simulink model "MICRORRED"  (R2018a)
settings: Solver=FixedStepDiscrete  StartTime=0.0  StopTime=0.7  FixedStep=1/(60*32)  RelTol=1e-3  EnableMultiTasking=on
InitFcn:
  | close
  | clear
  | clc
  | Ts=1/(60*32);
  | run script_client_3_inicio_ti.m
  | set_param('MICRORRED/EMISOR-RECEPTOR/TCP_IP_RX3/ESCRITURA', 'Value','0');
  | set_param('MICRORRED/EMISOR-RECEPTOR/TCP_IP_RX3/RETARDO', 'Value','0');
StopFcn:
  | %run script_graficas.m
undefined symbols (not defined in the file or in its folder): DiscIntNeverNeededParam, Int, Ip1, man, Vuc
libraries: powerlib x15, simulink x6, libreria_medidores3 x2, libreria_comunicaciones_red3 x1
(part 2 of 2)

== system MICRORRED/Carga 1 ==
  500 kw3 : powerlib/Elements/Three-Phase Parallel RLC Load  LConnTagsString=A|B|C  Configuration=Y (grounded)  NominalVoltage=13200  Vabc=[1e3 1e3 1e3]  Vabcp=[1e3 1e3 1e3]  NominalFrequency=60  UnbalancedPower=off  ActivePower=500e3  InductivePower=100e3  CapacitivePower=0  Pabc=[10e3 9e3 11e3]  QLabc=[100 90 110]  QCabc=[100 90 110]  Pabcp=[10e3 9e3 11e3]  QLabcp=[100 90 110]  QCabcp=[100 90 110]  Measurements=None  LoadType=constant Z
  a : PMIOPort  Side=Left
  b : PMIOPort  Port=2  Side=Left
  c : PMIOPort  Port=3  Side=Left
  connections:
  500 kw3/LConn1 -- a/RConn1
  500 kw3/LConn3 -- c/RConn1
  500 kw3/LConn2 -- b/RConn1

== system MICRORRED/Carga 2 ==
  500 kw3 : powerlib/Elements/Three-Phase Parallel RLC Load  LConnTagsString=A|B|C  Configuration=Y (grounded)  NominalVoltage=13200  Vabc=[1e3 1e3 1e3]  Vabcp=[1e3 1e3 1e3]  NominalFrequency=60  UnbalancedPower=off  ActivePower=500e3  InductivePower=100e3  CapacitivePower=0  Pabc=[10e3 9e3 11e3]  QLabc=[100 90 110]  QCabc=[100 90 110]  Pabcp=[10e3 9e3 11e3]  QLabcp=[100 90 110]  QCabcp=[100 90 110]  Measurements=None  LoadType=constant Z
  a : PMIOPort  Side=Left
  b : PMIOPort  Port=2  Side=Left
  c : PMIOPort  Port=3  Side=Left
  connections:
  500 kw3/LConn3 -- c/RConn1
  500 kw3/LConn2 -- b/RConn1
  a/RConn1 -- 500 kw3/LConn1

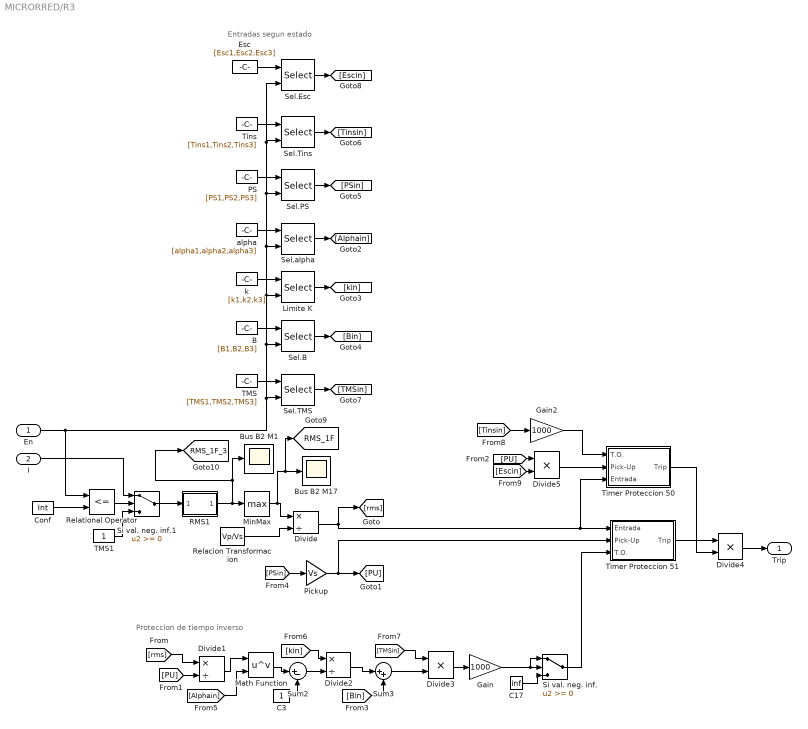
== system MICRORRED/R3 ==
  note: Proteccion de tiempo inverso
  note: Entradas segun estado
  En : Inport
  I : Inport  Port=2
  B : Constant  Value=[B1,B2,B3]
  Bus B2 M1 : Scope
  Bus B2 M17 : Scope
  C17 : Constant  Value=inf
  C3 : Constant
  Conf : Constant  Value=Int
  Divide : Product  Inputs=*/
  Divide1 : Product  Inputs=*/
  Divide2 : Product  Inputs=*/
  Divide3 : Product  Inputs=**
  Divide4 : Product  Inputs=**
  Divide5 : Product  Inputs=**
  Esc : Constant  Value=[Esc1,Esc2,Esc3]
  Gain : Gain  Gain=1000
  Gain2 : Gain  Gain=1000
  Limite K : Selector  InputPortWidth=3  IndexOptions=Index vector (port)  Indices=[1 2 3]  OutputSizes=1
  Math Function : Math  Operator=pow  SaturateOnIntegerOverflow=on
  MinMax : MinMax  Function=max
  PS : Constant  Value=[PS1,PS2,PS3]
  Pickup : Gain  Gain=Vs
  RMS1 : Subsystem
  Relacion Transformacion : Constant  Value=Vp/Vs
  Relational Operator : RelationalOperator  Operator=<=  OutDataTypeStr=boolean  RndMeth=Simplest
  Sel.B : Selector  InputPortWidth=3  IndexOptions=Index vector (port)  Indices=[1 2 3]  OutputSizes=1
  Sel.Esc : Selector  InputPortWidth=3  IndexOptions=Index vector (port)  Indices=[1 2 3]  OutputSizes=1
  Sel.PS : Selector  InputPortWidth=3  IndexOptions=Index vector (port)  Indices=[1 2 3]  OutputSizes=1
  Sel.TMS : Selector  InputPortWidth=3  IndexOptions=Index vector (port)  Indices=[1 2 3]  OutputSizes=1
  Sel.Tins : Selector  InputPortWidth=3  IndexOptions=Index vector (port)  Indices=[1 2 3]  OutputSizes=1
  Sel.alpha : Selector  InputPortWidth=3  IndexOptions=Index vector (port)  Indices=[1 2 3]  OutputSizes=1
  Si val. neg. inf. : Switch
  Si val. neg. inf.1 : Switch
  Sum2 : Sum  Inputs=|+-
  Sum3 : Sum  Inputs=|++
  TMS : Constant  Value=[TMS1,TMS2,TMS3]
  TMS1 : Constant
  Timer Proteccion 50 : Subsystem
  Timer Proteccion 51 : Subsystem
  Tins : Constant  Value=[Tins1,Tins2,Tins3]
  alpha : Constant  Value=[alpha1,alpha2,alpha3]
  k : Constant  Value=[k1,k2,k3]
  Trip : Outport
  tag scope: RMS_1F=global, RMS_1F_3=global
  wires:
  En/1 -> Relational Operator/1, Sel.TMS/2, Sel.B/2, Limite K/2, Sel.alpha/2, Sel.PS/2, Sel.Tins/2, Sel.Esc/2
  Divide4/1 -> Trip/1
  Tins/1 -> Sel.Tins/1
  [Escin] -> Divide5/2
  Sel.Esc/1 -> [Escin]
  C17/1 -> Si val. neg. inf./3
  Esc/1 -> Sel.Esc/1
  Math Function/1 -> Sum2/1
  [kin] -> Divide2/1
  Timer Proteccion 50/1(Trip) -> Divide4/2
  [PSin] -> Pickup/1
  Si val. neg. inf./1 -> Timer Proteccion 51/3(T.O.)
  Sel.TMS/1 -> [TMSin]
  PS/1 -> Sel.PS/1
  [Tinsin] -> Gain2/1
  Timer Proteccion 51/1(Trip) -> Divide4/1
  [Alphain] -> Math Function/2
  Divide3/1 -> Gain/1
  [PU] -> Divide1/2
  [PU] -> Divide5/1
  B/1 -> Sel.B/1
  Divide5/1 -> Timer Proteccion 50/2(Pick-Up)
  Divide2/1 -> Sum3/1
  Gain2/1 -> Timer Proteccion 50/1(T.O.)
  Gain/1 -> Si val. neg. inf./1, Si val. neg. inf./2
  Sum3/1 -> Divide3/2
  Sel.alpha/1 -> [Alphain]
  [Bin] -> Sum3/2
  Relacion Transformacion/1 -> Divide/2
  Divide/1 -> Timer Proteccion 51/1(Entrada), Timer Proteccion 50/3(Entrada), [rms]
  Sum2/1 -> Divide2/2
  Divide1/1 -> Math Function/1
  Limite K/1 -> [kin]
  [rms] -> Divide1/1
  Pickup/1 -> Timer Proteccion 51/2(Pick-Up), [PU]
  Sel.B/1 -> [Bin]
  Sel.PS/1 -> [PSin]
  MinMax/1 -> [RMS_1F], Bus B2 M17/1, Divide/1
  RMS1/1(Out1) -> [RMS_1F_3], Bus B2 M1/1, MinMax/1
  [TMSin] -> Divide3/1
  TMS/1 -> Sel.TMS/1
  C3/1 -> Sum2/2
  k/1 -> Limite K/1
  alpha/1 -> Sel.alpha/1
  Sel.Tins/1 -> [Tinsin]
  I/1 -> Si val. neg. inf.1/1
  Relational Operator/1 -> Si val. neg. inf.1/2
  Si val. neg. inf.1/1 -> RMS1/1(In1)
  Conf/1 -> Relational Operator/2
  TMS1/1 -> Si val. neg. inf.1/3

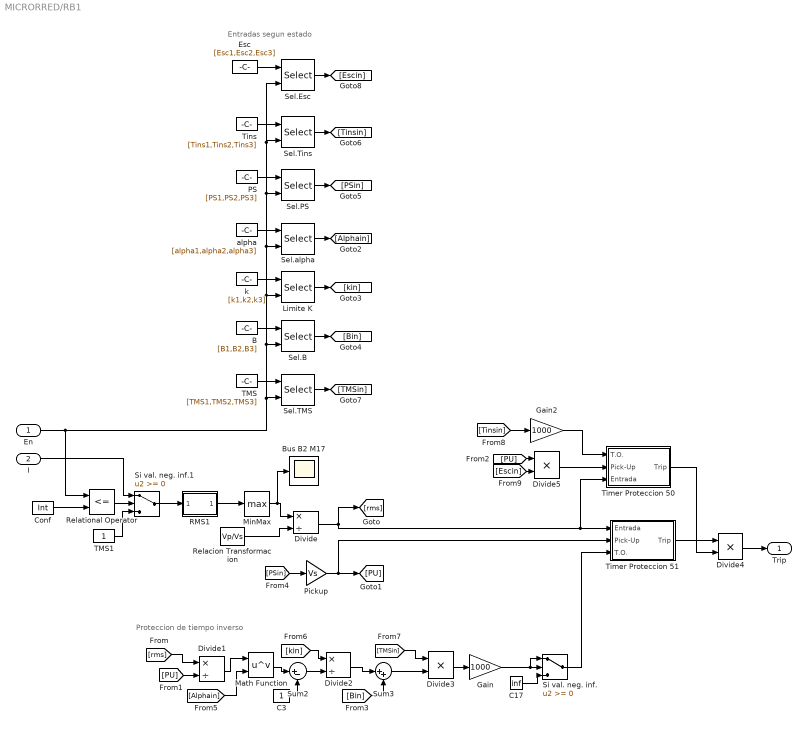
== system MICRORRED/RB1 ==
  note: Entradas segun estado
  note: Proteccion de tiempo inverso
  En : Inport
  I : Inport  Port=2
  B : Constant  Value=[B1,B2,B3]
  Bus B2 M17 : Scope
  C17 : Constant  Value=inf
  C3 : Constant
  Conf : Constant  Value=Int
  Divide : Product  Inputs=*/
  Divide1 : Product  Inputs=*/
  Divide2 : Product  Inputs=*/
  Divide3 : Product  Inputs=**
  Divide4 : Product  Inputs=**
  Divide5 : Product  Inputs=**
  Esc : Constant  Value=[Esc1,Esc2,Esc3]
  Gain : Gain  Gain=1000
  Gain2 : Gain  Gain=1000
  Limite K : Selector  InputPortWidth=3  IndexOptions=Index vector (port)  Indices=[1 2 3]  OutputSizes=1
  Math Function : Math  Operator=pow  SaturateOnIntegerOverflow=on
  MinMax : MinMax  Function=max
  PS : Constant  Value=[PS1,PS2,PS3]
  Pickup : Gain  Gain=Vs
  RMS1 : Subsystem
  Relacion Transformacion : Constant  Value=Vp/Vs
  Relational Operator : RelationalOperator  Operator=<=  OutDataTypeStr=boolean  RndMeth=Simplest
  Sel.B : Selector  InputPortWidth=3  IndexOptions=Index vector (port)  Indices=[1 2 3]  OutputSizes=1
  Sel.Esc : Selector  InputPortWidth=3  IndexOptions=Index vector (port)  Indices=[1 2 3]  OutputSizes=1
  Sel.PS : Selector  InputPortWidth=3  IndexOptions=Index vector (port)  Indices=[1 2 3]  OutputSizes=1
  Sel.TMS : Selector  InputPortWidth=3  IndexOptions=Index vector (port)  Indices=[1 2 3]  OutputSizes=1
  Sel.Tins : Selector  InputPortWidth=3  IndexOptions=Index vector (port)  Indices=[1 2 3]  OutputSizes=1
  Sel.alpha : Selector  InputPortWidth=3  IndexOptions=Index vector (port)  Indices=[1 2 3]  OutputSizes=1
  Si val. neg. inf. : Switch
  Si val. neg. inf.1 : Switch
  Sum2 : Sum  Inputs=|+-
  Sum3 : Sum  Inputs=|++
  TMS : Constant  Value=[TMS1,TMS2,TMS3]
  TMS1 : Constant
  Timer Proteccion 50 : Subsystem
  Timer Proteccion 51 : Subsystem
  Tins : Constant  Value=[Tins1,Tins2,Tins3]
  alpha : Constant  Value=[alpha1,alpha2,alpha3]
  k : Constant  Value=[k1,k2,k3]
  Trip : Outport
  wires:
  TMS1/1 -> Si val. neg. inf.1/3
  Conf/1 -> Relational Operator/2
  Si val. neg. inf.1/1 -> RMS1/1(In1)
  Relational Operator/1 -> Si val. neg. inf.1/2
  I/1 -> Si val. neg. inf.1/1
  Sel.Tins/1 -> [Tinsin]
  alpha/1 -> Sel.alpha/1
  k/1 -> Limite K/1
  C3/1 -> Sum2/2
  TMS/1 -> Sel.TMS/1
  [TMSin] -> Divide3/1
  RMS1/1(Out1) -> MinMax/1
  MinMax/1 -> Divide/1, Bus B2 M17/1
  Sel.PS/1 -> [PSin]
  Sel.B/1 -> [Bin]
  Pickup/1 -> [PU], Timer Proteccion 51/2(Pick-Up)
  [rms] -> Divide1/1
  Limite K/1 -> [kin]
  Divide1/1 -> Math Function/1
  Sum2/1 -> Divide2/2
  Divide/1 -> [rms], Timer Proteccion 50/3(Entrada), Timer Proteccion 51/1(Entrada)
  Relacion Transformacion/1 -> Divide/2
  [Bin] -> Sum3/2
  Sel.alpha/1 -> [Alphain]
  Sum3/1 -> Divide3/2
  Gain/1 -> Si val. neg. inf./2, Si val. neg. inf./1
  Gain2/1 -> Timer Proteccion 50/1(T.O.)
  Divide2/1 -> Sum3/1
  Divide5/1 -> Timer Proteccion 50/2(Pick-Up)
  B/1 -> Sel.B/1
  [PU] -> Divide5/1
  [PU] -> Divide1/2
  Divide3/1 -> Gain/1
  [Alphain] -> Math Function/2
  Timer Proteccion 51/1(Trip) -> Divide4/1
  [Tinsin] -> Gain2/1
  PS/1 -> Sel.PS/1
  Sel.TMS/1 -> [TMSin]
  Si val. neg. inf./1 -> Timer Proteccion 51/3(T.O.)
  [PSin] -> Pickup/1
  Timer Proteccion 50/1(Trip) -> Divide4/2
  [kin] -> Divide2/1
  Math Function/1 -> Sum2/1
  Esc/1 -> Sel.Esc/1
  C17/1 -> Si val. neg. inf./3
  Sel.Esc/1 -> [Escin]
  [Escin] -> Divide5/2
  Tins/1 -> Sel.Tins/1
  Divide4/1 -> Trip/1
  En/1 -> Sel.Esc/2, Sel.Tins/2, Sel.PS/2, Sel.alpha/2, Limite K/2, Sel.B/2, Sel.TMS/2, Relational Operator/1

== system MICRORRED/Subsystem ==
  Trigger : TriggerPort  VariantControl=Variant  ShowOutputPort=on  OutputDataType=double  InitialTriggerSignalState=positive  PortDimensions=1
  Display : Display
  Out1 : Outport
  wires:
  Trigger/1 -> Display/1, Out1/1

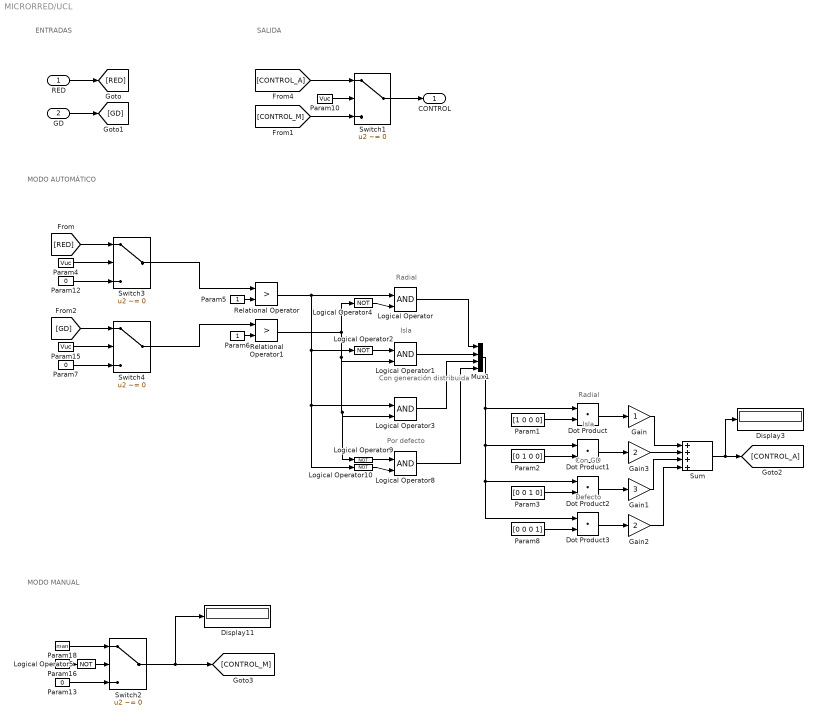
== system MICRORRED/UCL ==
  note: ENTRADAS
  note: Con generación
      | distribuida
  note: Isla
  note: Radial
  note: SALIDA
  note: MODO AUTOMÁTICO
  note: MODO MANUAL
  note: Radial
  note: Isla
  note: Con GD
  note: Por defecto
  note: Defecto
  RED : Inport
  GD : Inport  Port=2
  Display11 : Display
  Display3 : Display
  Dot Product{,1..3} (4 alike) : DotProduct  InputSameDT=on  OutDataTypeStr=Inherit: Inherit via internal rule
  Gain : Gain
  Gain1 : Gain  Gain=3
  Gain2 : Gain  Gain=2
  Gain3 : Gain  Gain=2
  Logical Operator{,1,3,8} (4 alike) : Logic  IconShape=distinctive  AllPortsSameDT=off  OutDataTypeStr=boolean
  Logical Operator{2,4..5,9..10} (5 alike) : Logic  Operator=NOT  AllPortsSameDT=off  OutDataTypeStr=boolean
  Mux1 : Mux
  Param1 : Constant  Value=[1 0 0 0]  OutDataTypeStr=boolean
  Param{4,10,15..16} (4 alike) : Constant  Value=Vuc
  Param12 : Constant  Value=0
  Param13 : Constant  Value=0
  Param18 : Constant  Value=man
  Param2 : Constant  Value=[0 1 0 0]  OutDataTypeStr=boolean
  Param3 : Constant  Value=[0 0 1 0]  OutDataTypeStr=boolean
  Param5 : Constant
  Param6 : Constant
  Param7 : Constant  Value=0
  Param8 : Constant  Value=[0 0 0 1]  OutDataTypeStr=boolean
  Relational Operator : RelationalOperator  Operator=>  OutDataTypeStr=boolean  RndMeth=Nearest
  Relational Operator1 : RelationalOperator  Operator=>  OutDataTypeStr=boolean  RndMeth=Nearest
  Sum : Sum  Inputs=+|+|+|+
  Switch{1..4} (4 alike) : Switch  Criteria=u2 ~= 0
  CONTROL : Outport
  wires:
  Relational Operator/1 -> Logical Operator10/1, Logical Operator3/1, Logical Operator2/1, Logical Operator/1
  Param6/1 -> Relational Operator1/2
  Param5/1 -> Relational Operator/2
  Logical Operator2/1 -> Logical Operator1/1
  Logical Operator4/1 -> Logical Operator/2
  Logical Operator/1 -> Mux1/1
  Logical Operator1/1 -> Mux1/2
  Logical Operator3/1 -> Mux1/3
  Param1/1 -> Dot Product/2
  Dot Product/1 -> Gain/1
  Param2/1 -> Dot Product1/2
  Param3/1 -> Dot Product2/2
  Dot Product1/1 -> Gain3/1
  Dot Product2/1 -> Gain1/1
  Gain/1 -> Sum/1
  Logical Operator5/1 -> Switch2/2
  RED/1 -> [RED]
  Param18/1 -> Switch2/1
  GD/1 -> [GD]
  [RED] -> Switch3/1
  Param12/1 -> Switch3/3
  [GD] -> Switch4/1
  Param7/1 -> Switch4/3
  Param13/1 -> Switch2/3
  Param4/1 -> Switch3/2
  Param15/1 -> Switch4/2
  Param16/1 -> Logical Operator5/1
  Switch2/1 -> [CONTROL_M], Display11/1
  Gain3/1 -> Sum/2
  Gain1/1 -> Sum/3
  Sum/1 -> [CONTROL_A], Display3/1
  Switch3/1 -> Relational Operator/1
  Switch4/1 -> Relational Operator1/1
  Logical Operator9/1 -> Logical Operator8/1
  Logical Operator10/1 -> Logical Operator8/2
  Relational Operator1/1 -> Logical Operator4/1, Logical Operator9/1, Logical Operator3/2, Logical Operator1/2
  Logical Operator8/1 -> Mux1/4
  Param8/1 -> Dot Product3/2
  Mux1/1 -> Dot Product3/1, Dot Product2/1, Dot Product1/1, Dot Product/1
  Dot Product3/1 -> Gain2/1
  Gain2/1 -> Sum/4
  [CONTROL_A] -> Switch1/1
  [CONTROL_M] -> Switch1/3
  Param10/1 -> Switch1/2
  Switch1/1 -> CONTROL/1

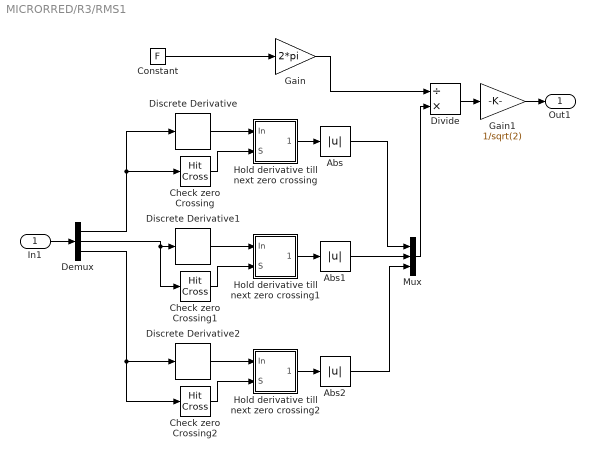
== system MICRORRED/R3/RMS1 ==
  In1 : Inport
  Abs : Abs
  Abs1 : Abs
  Abs2 : Abs
  Check zero Crossing : HitCross
  Check zero Crossing1 : HitCross
  Check zero Crossing2 : HitCross
  Constant : Constant  Value=F
  Demux : Demux  Outputs=3
  Discrete Derivative : simulink/Discrete/Discrete Derivative  gainval=1.0  ICPrevScaledInput=0.0  OutMin=[]  OutMax=[]  OutDataType=fixdt(1, 16)  OutScaling=2^-10  DoSatur=off
  Discrete Derivative1 : simulink/Discrete/Discrete Derivative  gainval=1.0  ICPrevScaledInput=0.0  OutMin=[]  OutMax=[]  OutDataType=fixdt(1, 16)  OutScaling=2^-10  DoSatur=off
  Discrete Derivative2 : simulink/Discrete/Discrete Derivative  gainval=1.0  ICPrevScaledInput=0.0  OutMin=[]  OutMax=[]  OutDataType=fixdt(1, 16)  OutScaling=2^-10  DoSatur=off
  Divide : Product  Inputs=/*
  Gain : Gain  Gain=2*pi
  Gain1 : Gain  Gain=1/sqrt(2)
  Hold derivative till next zero crossing : Subsystem  AncestorBlock=|  DialogController=POWERSYS.PowerSysDialog  mask(Discrete Sample & Hold){ic=0, Ts=-1}
      | powerlib_extras/Discrete 
      | Control Blocks/Discrete
      | Sample & Hold
      mask prompts: ic "Initial condition:"; Ts "Sample time:"
      mask help: The output follows input 1 (In) as long as input 2 (S) is TRUE (1) . The output is held when input 2 becomes FALSE (0). The output initial value is specified by the parameter "Initial condition".
      mask init:
      | power_initmask();
      mask Help: This block is part of a subset of blocks in the Extras library that does not have documentation associated with it, other than the block mask description.
      mask Display: disp('S/H')
  Hold derivative till next zero crossing1 : Subsystem  AncestorBlock=|  DialogController=POWERSYS.PowerSysDialog  mask(Discrete Sample & Hold){ic=0, Ts=-1}
      | powerlib_extras/Discrete 
      | Control Blocks/Discrete
      | Sample & Hold
      mask prompts: ic "Initial condition:"; Ts "Sample time:"
      mask help: The output follows input 1 (In) as long as input 2 (S) is TRUE (1) . The output is held when input 2 becomes FALSE (0). The output initial value is specified by the parameter "Initial condition".
      mask init:
      | power_initmask();
      mask Help: This block is part of a subset of blocks in the Extras library that does not have documentation associated with it, other than the block mask description.
      mask Display: disp('S/H')
  Hold derivative till next zero crossing2 : Subsystem  AncestorBlock=|  DialogController=POWERSYS.PowerSysDialog  mask(Discrete Sample & Hold){ic=0, Ts=-1}
      | powerlib_extras/Discrete 
      | Control Blocks/Discrete
      | Sample & Hold
      mask prompts: ic "Initial condition:"; Ts "Sample time:"
      mask help: The output follows input 1 (In) as long as input 2 (S) is TRUE (1) . The output is held when input 2 becomes FALSE (0). The output initial value is specified by the parameter "Initial condition".
      mask init:
      | power_initmask();
      mask Help: This block is part of a subset of blocks in the Extras library that does not have documentation associated with it, other than the block mask description.
      mask Display: disp('S/H')
  Mux : Mux  Inputs=3
  Out1 : Outport
  wires:
  Discrete Derivative/1 -> Hold derivative till next zero crossing/1(In)
  Check zero Crossing/1 -> Hold derivative till next zero crossing/2(S)
  Hold derivative till next zero crossing/1("   ") -> Abs/1
  Constant/1 -> Gain/1
  Gain/1 -> Divide/1
  Abs/1 -> Mux/1
  Demux/1 -> Check zero Crossing/1, Discrete Derivative/1
  Divide/1 -> Gain1/1
  Gain1/1 -> Out1/1
  Hold derivative till next zero crossing1/1("   ") -> Abs1/1
  Check zero Crossing1/1 -> Hold derivative till next zero crossing1/2(S)
  Discrete Derivative1/1 -> Hold derivative till next zero crossing1/1(In)
  Discrete Derivative2/1 -> Hold derivative till next zero crossing2/1(In)
  Check zero Crossing2/1 -> Hold derivative till next zero crossing2/2(S)
  Hold derivative till next zero crossing2/1("   ") -> Abs2/1
  Demux/2 -> Check zero Crossing1/1, Discrete Derivative1/1
  Demux/3 -> Check zero Crossing2/1, Discrete Derivative2/1
  Abs1/1 -> Mux/2
  Mux/1 -> Divide/2
  Abs2/1 -> Mux/3
  In1/1 -> Demux/1

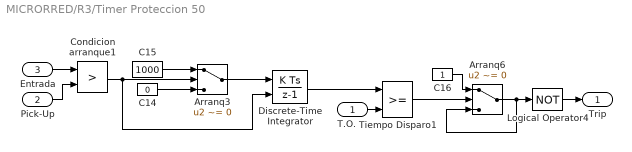
== system MICRORRED/R3/Timer Proteccion 50 ==
  T.O. : Inport
  Pick-Up : Inport  Port=2
  Entrada : Inport  Port=3
  Arranq3 : Switch  Criteria=u2 ~= 0  Threshold=Ip1
  Arranq6 : Switch  Criteria=u2 ~= 0  Threshold=Ip1  ZeroCross=off
  C14 : Constant  Value=0
  C15 : Constant  Value=1000
  C16 : Constant
  Condicion arranque1 : RelationalOperator  Operator=>  OutDataTypeStr=boolean  RndMeth=Nearest
  Discrete-Time Integrator : DiscreteIntegrator  ExternalReset=falling  SampleTime=-1  ICPrevOutput=DiscIntNeverNeededParam  ICPrevScaledInput=DiscIntNeverNeededParam
  Logical Operator4 : Logic  Operator=NOT  AllPortsSameDT=off  OutDataTypeStr=boolean
  Tiempo Disparo1 : RelationalOperator  OutDataTypeStr=boolean  RndMeth=Nearest
  Trip : Outport
  wires:
  C16/1 -> Arranq6/1
  Arranq6/1 -> Logical Operator4/1, Arranq6/3
  Tiempo Disparo1/1 -> Arranq6/2
  C15/1 -> Arranq3/1
  C14/1 -> Arranq3/3
  Arranq3/1 -> Discrete-Time Integrator/1
  Condicion arranque1/1 -> Arranq3/2, Discrete-Time Integrator/2
  Pick-Up/1 -> Condicion arranque1/2
  Discrete-Time Integrator/1 -> Tiempo Disparo1/1
  Logical Operator4/1 -> Trip/1
  Entrada/1 -> Condicion arranque1/1
  T.O./1 -> Tiempo Disparo1/2

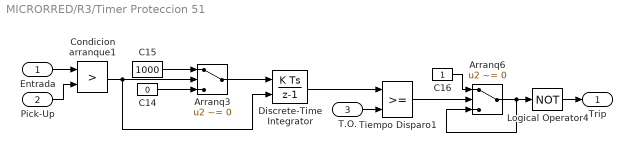
== system MICRORRED/R3/Timer Proteccion 51 ==
  Entrada : Inport
  Pick-Up : Inport  Port=2
  T.O. : Inport  Port=3
  Arranq3 : Switch  Criteria=u2 ~= 0  Threshold=Ip1
  Arranq6 : Switch  Criteria=u2 ~= 0  Threshold=Ip1  ZeroCross=off
  C14 : Constant  Value=0
  C15 : Constant  Value=1000
  C16 : Constant
  Condicion arranque1 : RelationalOperator  Operator=>  OutDataTypeStr=boolean  RndMeth=Nearest
  Discrete-Time Integrator : DiscreteIntegrator  ExternalReset=falling  SampleTime=-1  ICPrevOutput=DiscIntNeverNeededParam  ICPrevScaledInput=DiscIntNeverNeededParam
  Logical Operator4 : Logic  Operator=NOT  AllPortsSameDT=off  OutDataTypeStr=boolean
  Tiempo Disparo1 : RelationalOperator  OutDataTypeStr=boolean  RndMeth=Nearest
  Trip : Outport
  wires:
  C16/1 -> Arranq6/1
  Arranq6/1 -> Logical Operator4/1, Arranq6/3
  Tiempo Disparo1/1 -> Arranq6/2
  T.O./1 -> Tiempo Disparo1/2
  C15/1 -> Arranq3/1
  C14/1 -> Arranq3/3
  Arranq3/1 -> Discrete-Time Integrator/1
  Condicion arranque1/1 -> Arranq3/2, Discrete-Time Integrator/2
  Pick-Up/1 -> Condicion arranque1/2
  Entrada/1 -> Condicion arranque1/1
  Discrete-Time Integrator/1 -> Tiempo Disparo1/1
  Logical Operator4/1 -> Trip/1

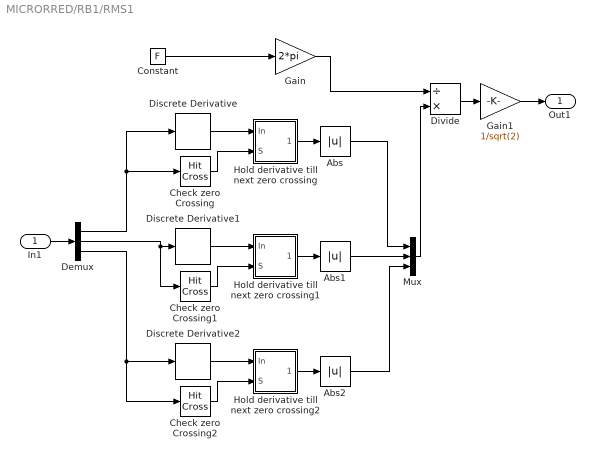
== system MICRORRED/RB1/RMS1 ==
  In1 : Inport
  Abs : Abs
  Abs1 : Abs
  Abs2 : Abs
  Check zero Crossing : HitCross
  Check zero Crossing1 : HitCross
  Check zero Crossing2 : HitCross
  Constant : Constant  Value=F
  Demux : Demux  Outputs=3
  Discrete Derivative : simulink/Discrete/Discrete Derivative  gainval=1.0  ICPrevScaledInput=0.0  OutMin=[]  OutMax=[]  OutDataType=fixdt(1, 16)  OutScaling=2^-10  DoSatur=off
  Discrete Derivative1 : simulink/Discrete/Discrete Derivative  gainval=1.0  ICPrevScaledInput=0.0  OutMin=[]  OutMax=[]  OutDataType=fixdt(1, 16)  OutScaling=2^-10  DoSatur=off
  Discrete Derivative2 : simulink/Discrete/Discrete Derivative  gainval=1.0  ICPrevScaledInput=0.0  OutMin=[]  OutMax=[]  OutDataType=fixdt(1, 16)  OutScaling=2^-10  DoSatur=off
  Divide : Product  Inputs=/*
  Gain : Gain  Gain=2*pi
  Gain1 : Gain  Gain=1/sqrt(2)
  Hold derivative till next zero crossing : Subsystem  AncestorBlock=|  DialogController=POWERSYS.PowerSysDialog  mask(Discrete Sample & Hold){ic=0, Ts=-1}
      | powerlib_extras/Discrete 
      | Control Blocks/Discrete
      | Sample & Hold
      mask prompts: ic "Initial condition:"; Ts "Sample time:"
      mask help: The output follows input 1 (In) as long as input 2 (S) is TRUE (1) . The output is held when input 2 becomes FALSE (0). The output initial value is specified by the parameter "Initial condition".
      mask init:
      | power_initmask();
      mask Help: This block is part of a subset of blocks in the Extras library that does not have documentation associated with it, other than the block mask description.
      mask Display: disp('S/H')
  Hold derivative till next zero crossing1 : Subsystem  AncestorBlock=|  DialogController=POWERSYS.PowerSysDialog  mask(Discrete Sample & Hold){ic=0, Ts=-1}
      | powerlib_extras/Discrete 
      | Control Blocks/Discrete
      | Sample & Hold
      mask prompts: ic "Initial condition:"; Ts "Sample time:"
      mask help: The output follows input 1 (In) as long as input 2 (S) is TRUE (1) . The output is held when input 2 becomes FALSE (0). The output initial value is specified by the parameter "Initial condition".
      mask init:
      | power_initmask();
      mask Help: This block is part of a subset of blocks in the Extras library that does not have documentation associated with it, other than the block mask description.
      mask Display: disp('S/H')
  Hold derivative till next zero crossing2 : Subsystem  AncestorBlock=|  DialogController=POWERSYS.PowerSysDialog  mask(Discrete Sample & Hold){ic=0, Ts=-1}
      | powerlib_extras/Discrete 
      | Control Blocks/Discrete
      | Sample & Hold
      mask prompts: ic "Initial condition:"; Ts "Sample time:"
      mask help: The output follows input 1 (In) as long as input 2 (S) is TRUE (1) . The output is held when input 2 becomes FALSE (0). The output initial value is specified by the parameter "Initial condition".
      mask init:
      | power_initmask();
      mask Help: This block is part of a subset of blocks in the Extras library that does not have documentation associated with it, other than the block mask description.
      mask Display: disp('S/H')
  Mux : Mux  Inputs=3
  Out1 : Outport
  wires:
  In1/1 -> Demux/1
  Abs2/1 -> Mux/3
  Mux/1 -> Divide/2
  Abs1/1 -> Mux/2
  Demux/3 -> Discrete Derivative2/1, Check zero Crossing2/1
  Demux/2 -> Discrete Derivative1/1, Check zero Crossing1/1
  Hold derivative till next zero crossing2/1("   ") -> Abs2/1
  Check zero Crossing2/1 -> Hold derivative till next zero crossing2/2(S)
  Discrete Derivative2/1 -> Hold derivative till next zero crossing2/1(In)
  Discrete Derivative1/1 -> Hold derivative till next zero crossing1/1(In)
  Check zero Crossing1/1 -> Hold derivative till next zero crossing1/2(S)
  Hold derivative till next zero crossing1/1("   ") -> Abs1/1
  Gain1/1 -> Out1/1
  Divide/1 -> Gain1/1
  Demux/1 -> Discrete Derivative/1, Check zero Crossing/1
  Abs/1 -> Mux/1
  Gain/1 -> Divide/1
  Constant/1 -> Gain/1
  Hold derivative till next zero crossing/1("   ") -> Abs/1
  Check zero Crossing/1 -> Hold derivative till next zero crossing/2(S)
  Discrete Derivative/1 -> Hold derivative till next zero crossing/1(In)

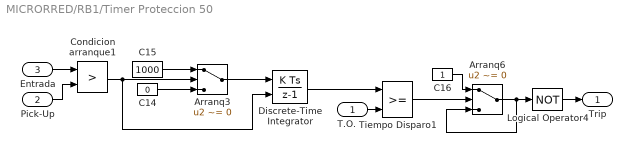
== system MICRORRED/RB1/Timer Proteccion 50 ==
  T.O. : Inport
  Pick-Up : Inport  Port=2
  Entrada : Inport  Port=3
  Arranq3 : Switch  Criteria=u2 ~= 0  Threshold=Ip1
  Arranq6 : Switch  Criteria=u2 ~= 0  Threshold=Ip1  ZeroCross=off
  C14 : Constant  Value=0
  C15 : Constant  Value=1000
  C16 : Constant
  Condicion arranque1 : RelationalOperator  Operator=>  OutDataTypeStr=boolean  RndMeth=Nearest
  Discrete-Time Integrator : DiscreteIntegrator  ExternalReset=falling  SampleTime=-1  ICPrevOutput=DiscIntNeverNeededParam  ICPrevScaledInput=DiscIntNeverNeededParam
  Logical Operator4 : Logic  Operator=NOT  AllPortsSameDT=off  OutDataTypeStr=boolean
  Tiempo Disparo1 : RelationalOperator  OutDataTypeStr=boolean  RndMeth=Nearest
  Trip : Outport
  wires:
  T.O./1 -> Tiempo Disparo1/2
  Entrada/1 -> Condicion arranque1/1
  Logical Operator4/1 -> Trip/1
  Discrete-Time Integrator/1 -> Tiempo Disparo1/1
  Pick-Up/1 -> Condicion arranque1/2
  Condicion arranque1/1 -> Discrete-Time Integrator/2, Arranq3/2
  Arranq3/1 -> Discrete-Time Integrator/1
  C14/1 -> Arranq3/3
  C15/1 -> Arranq3/1
  Tiempo Disparo1/1 -> Arranq6/2
  Arranq6/1 -> Arranq6/3, Logical Operator4/1
  C16/1 -> Arranq6/1

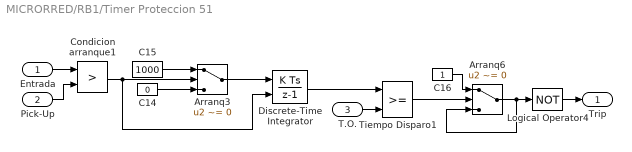
== system MICRORRED/RB1/Timer Proteccion 51 ==
  Entrada : Inport
  Pick-Up : Inport  Port=2
  T.O. : Inport  Port=3
  Arranq3 : Switch  Criteria=u2 ~= 0  Threshold=Ip1
  Arranq6 : Switch  Criteria=u2 ~= 0  Threshold=Ip1  ZeroCross=off
  C14 : Constant  Value=0
  C15 : Constant  Value=1000
  C16 : Constant
  Condicion arranque1 : RelationalOperator  Operator=>  OutDataTypeStr=boolean  RndMeth=Nearest
  Discrete-Time Integrator : DiscreteIntegrator  ExternalReset=falling  SampleTime=-1  ICPrevOutput=DiscIntNeverNeededParam  ICPrevScaledInput=DiscIntNeverNeededParam
  Logical Operator4 : Logic  Operator=NOT  AllPortsSameDT=off  OutDataTypeStr=boolean
  Tiempo Disparo1 : RelationalOperator  OutDataTypeStr=boolean  RndMeth=Nearest
  Trip : Outport
  wires:
  Logical Operator4/1 -> Trip/1
  Discrete-Time Integrator/1 -> Tiempo Disparo1/1
  Entrada/1 -> Condicion arranque1/1
  Pick-Up/1 -> Condicion arranque1/2
  Condicion arranque1/1 -> Discrete-Time Integrator/2, Arranq3/2
  Arranq3/1 -> Discrete-Time Integrator/1
  C14/1 -> Arranq3/3
  C15/1 -> Arranq3/1
  T.O./1 -> Tiempo Disparo1/2
  Tiempo Disparo1/1 -> Arranq6/2
  Arranq6/1 -> Arranq6/3, Logical Operator4/1
  C16/1 -> Arranq6/1

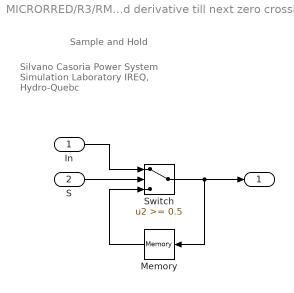
== system MICRORRED/R3/RMS1/Hold derivative till next zero crossing ==
  note: Silvano Casoria
      | Power System Simulation Laboratory
      | IREQ, Hydro-Quebc
  note: Sample and Hold
  In : Inport
  S : Inport  Port=2
  Memory : Memory
  Switch : Switch  Threshold=0.5  SaturateOnIntegerOverflow=on  InputSameDT=on
  "   " : Outport  InitialOutput=0
  wires:
  S/1 -> Switch/2
  In/1 -> Switch/1
  Memory/1 -> Switch/3
  Switch/1 -> Memory/1, "   "/1

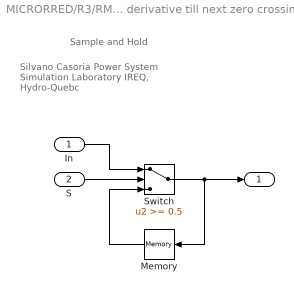
== system MICRORRED/R3/RMS1/Hold derivative till next zero crossing1 ==
  note: Sample and Hold
  note: Silvano Casoria
      | Power System Simulation Laboratory
      | IREQ, Hydro-Quebc
  In : Inport
  S : Inport  Port=2
  Memory : Memory
  Switch : Switch  Threshold=0.5  SaturateOnIntegerOverflow=on  InputSameDT=on
  "   " : Outport  InitialOutput=0
  wires:
  Switch/1 -> "   "/1, Memory/1
  Memory/1 -> Switch/3
  In/1 -> Switch/1
  S/1 -> Switch/2

== system MICRORRED/R3/RMS1/Hold derivative till next zero crossing2 ==
  note: Silvano Casoria
      | Power System Simulation Laboratory
      | IREQ, Hydro-Quebc
  note: Sample and Hold
  In : Inport
  S : Inport  Port=2
  Memory : Memory
  Switch : Switch  Threshold=0.5  SaturateOnIntegerOverflow=on  InputSameDT=on
  "   " : Outport  InitialOutput=0
  wires:
  S/1 -> Switch/2
  In/1 -> Switch/1
  Memory/1 -> Switch/3
  Switch/1 -> Memory/1, "   "/1

== system MICRORRED/RB1/RMS1/Hold derivative till next zero crossing ==
  note: Sample and Hold
  note: Silvano Casoria
      | Power System Simulation Laboratory
      | IREQ, Hydro-Quebc
  In : Inport
  S : Inport  Port=2
  Memory : Memory
  Switch : Switch  Threshold=0.5  SaturateOnIntegerOverflow=on  InputSameDT=on
  "   " : Outport  InitialOutput=0
  wires:
  Switch/1 -> "   "/1, Memory/1
  Memory/1 -> Switch/3
  In/1 -> Switch/1
  S/1 -> Switch/2

== system MICRORRED/RB1/RMS1/Hold derivative till next zero crossing1 ==
  note: Silvano Casoria
      | Power System Simulation Laboratory
      | IREQ, Hydro-Quebc
  note: Sample and Hold
  In : Inport
  S : Inport  Port=2
  Memory : Memory
  Switch : Switch  Threshold=0.5  SaturateOnIntegerOverflow=on  InputSameDT=on
  "   " : Outport  InitialOutput=0
  wires:
  S/1 -> Switch/2
  In/1 -> Switch/1
  Memory/1 -> Switch/3
  Switch/1 -> Memory/1, "   "/1

== system MICRORRED/RB1/RMS1/Hold derivative till next zero crossing2 ==
  note: Sample and Hold
  note: Silvano Casoria
      | Power System Simulation Laboratory
      | IREQ, Hydro-Quebc
  In : Inport
  S : Inport  Port=2
  Memory : Memory
  Switch : Switch  Threshold=0.5  SaturateOnIntegerOverflow=on  InputSameDT=on
  "   " : Outport  InitialOutput=0
  wires:
  Switch/1 -> "   "/1, Memory/1
  Memory/1 -> Switch/3
  In/1 -> Switch/1
  S/1 -> Switch/2
